simulink model "pll918"  (R2021b)
settings: Solver=VariableStepAuto  StartTime=0.0  StopTime=0.1  RelTol=1e-3
libraries: spsIGBTDiodeLib x6, cstextras x4, spsAlphaBetaZerotodq0Lib x3, slpidlib x3, spsabctoAlphaBetaZeroLib x3, spsThreePhaseSeriesRLCBranchLib x2, spsThreePhaseVIMeasurementLib x2, spsAlphaBetaZerotoabcLib x1, spsGroundLib x1, spsSawtoothGeneratorLib x1, spsDCVoltageSourceLib x1, spsSeriesRLCBranchLib x1
settings Model: Creator=Admin  LastModifiedBy=Admin

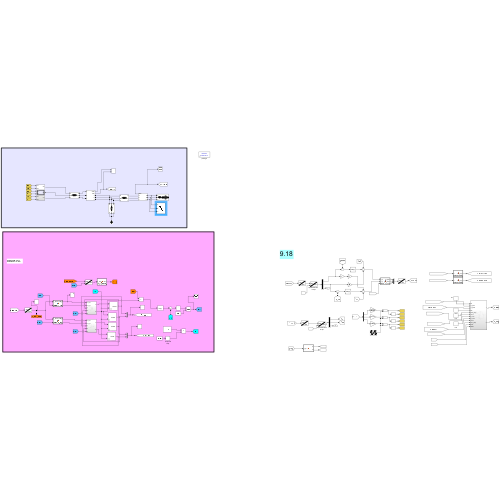
[thumbnail: Simulink's stored preview of the top-level diagram]
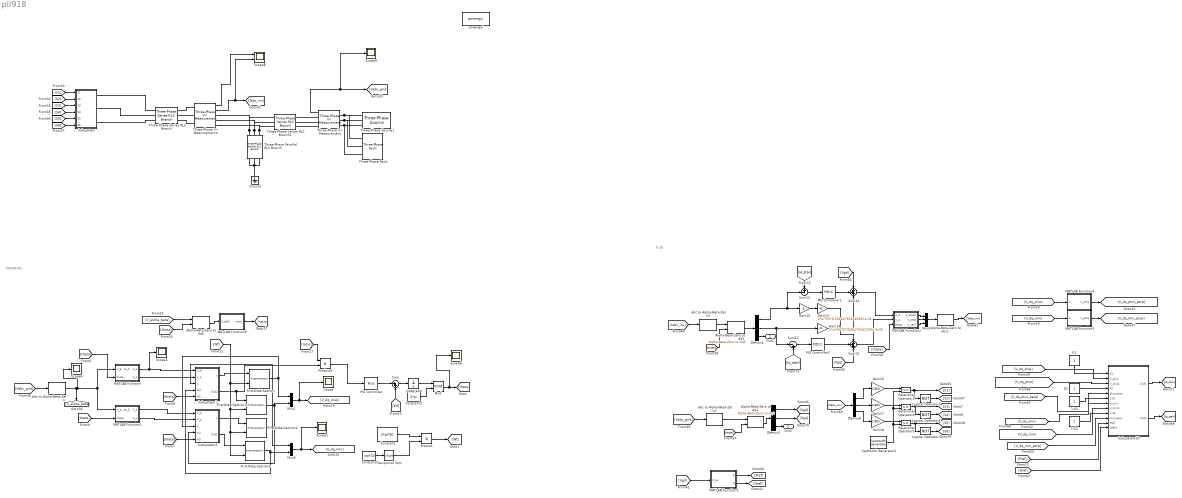
== system pll918 ==
  note: DDSRF-PLL
  note: 9.18
  1-K1 : Constant
  1-K2 : Constant
  Alpha-Beta-Zero to abc1 : spsAlphaBetaZerotoabcLib/Alpha-Beta-Zero to abc
      settings: SourceProductBaseCode=PS
  Alpha-Beta-Zero to dq0 : spsAlphaBetaZerotodq0Lib/Alpha-Beta-Zero to dq0  Alignment=90 degrees behind phase A axis
      settings: SourceProductBaseCode=PS
  Alpha-Beta-Zero to dq1 : spsAlphaBetaZerotodq0Lib/Alpha-Beta-Zero to dq0  Alignment=90 degrees behind phase A axis
      settings: SourceProductBaseCode=PS
  Alpha-Beta-Zero to dq2 : spsAlphaBetaZerotodq0Lib/Alpha-Beta-Zero to dq0  Alignment=90 degrees behind phase A axis
      settings: SourceProductBaseCode=PS
  Constant : Constant  Value=2*pi*50
  Constant1 : Constant  Value=sqrt(2)
  Constant2 : Constant  Value=2*pi
  Demux3 : Demux  Outputs=3
  Demux4 : Demux  Outputs=3
  Demux6 : Demux  Outputs=3
  FirstOrderSection{,1..3} (4 alike) : cstextras/FirstOrderSection  VariantControl=(default)
      settings: SourceProductBaseCode=CT
  Gain13 : Gain  Gain=2*pi*50*6.254627916220947e-05
  Gain14 : Gain  Gain=2*pi*50*6.254627916220947e-05
  Gain15 : Gain  Gain=-1
  Gain16 : Gain  Gain=2/800
  Gain17 : Gain  Gain=2/800
  Gain18 : Gain  Gain=2/800
  Ground : spsGroundLib/Ground  LConnTagsString=a
  Integrator : Integrator
  "K1 " : Constant
  K2 : Constant
  Logical Operator3 : Logic  Operator=NOT  AllPortsSameDT=off  OutDataTypeStr=boolean
  Logical Operator4 : Logic  Operator=NOT  AllPortsSameDT=off  OutDataTypeStr=boolean
  Logical Operator5 : Logic  Operator=NOT  AllPortsSameDT=off  OutDataTypeStr=boolean
  MATLAB Function : MATLAB Function  TreatAsAtomicUnit=on
  MATLAB Function1 : MATLAB Function  TreatAsAtomicUnit=on
  MATLAB Function2 : MATLAB Function  TreatAsAtomicUnit=on
  MATLAB Function3 : MATLAB Function  TreatAsAtomicUnit=on
  MATLAB Function4 : MATLAB Function  TreatAsAtomicUnit=on
  MATLAB Function5 : MATLAB Function  TreatAsAtomicUnit=on
  MATLAB Function8 : MATLAB Function  TreatAsAtomicUnit=on
  Mod : Math  Operator=mod  SaturateOnIntegerOverflow=on
  Mux1 : Mux  Inputs=2
  Mux3 : Mux  Inputs=3
  Mux6 : Mux  Inputs=2
  PID Controller : slpidlib/PID Controller  Controller=PI  Form=Parallel  TimeDomain=Continuous-time  UseExternalTs=off  SampleTime=-1  IntegratorMethod=Forward Euler  FilterMethod=Forward Euler  ControllerParametersSource=internal  P=222.1  I=9e-3  D=0  UseFilter=on  N=100  TunerSelectOption=Transfer Function Based (PID Tuner App)  InitialConditionSource=internal  InitialConditionForIntegrator=0  InitialConditionForFilter=0  DifferentiatorICPrevScaledInput=0  ExternalReset=none  TrackingMode=off  Kt=1  LimitOutput=off  SatLimitsSource=internal  UpperSaturationLimit=inf  LowerSaturationLimit=-inf  LinearizeAsGain=on  AntiWindupMode=none  Kb=1  POutMin=[]  POutMax=[]  IOutMin=[]  IOutMax=[]  DOutMin=[]  DOutMax=[]  NOutMin=[]  NOutMax=[]  SumOutMin=[]  SumOutMax=[]  SaturationOutMin=[]  SaturationOutMax=[]  PParamMin=[]  PParamMax=[]  IParamMin=[]  IParamMax=[]  DParamMin=[]  DParamMax=[]  NParamMin=[]  NParamMax=[]  KbParamMin=[]  KbParamMax=[]  KtParamMin=[]  KtParamMax=[]  KbOutMin=[]  KbOutMax=[]  KtOutMin=[]  KtOutMax=[]  IntegratorOutMin=[]  IntegratorOutMax=[]  FilterOutMin=[]  FilterOutMax=[]  SumI1OutMin=[]  SumI1OutMax=[]  SumI2OutMin=[]  SumI2OutMax=[]  SumI3OutMin=[]  SumI3OutMax=[]  SumI4OutMin=[]  SumI4OutMax=[]  SumDOutMin=[]  SumDOutMax=[]  DifferentiatorOutMin=[]  DifferentiatorOutMax=[]  FilterDiffOutCoefMin=[]  FilterDiffOutCoefMax=[]  ReciprocalOutMin=[]  ReciprocalOutMax=[]  SumDenOutMin=[]  SumDenOutMax=[]  SumNumOutMin=[]  SumNumOutMax=[]  DivideOutMin=[]  DivideOutMax=[]  UdiffTsProdOutMin=[]  UdiffTsProdOutMax=[]  NTsProdOutMin=[]  NTsProdOutMax=[]  UintegralTsProdOutMin=[]  UintegralTsProdOutMax=[]  UngainTsProdOutMin=[]  UngainTsProdOutMax=[]  FilterDenConstantOutDataTypeStr=Inherit: Inherit via back propagation  FilterDenConstantOutMin=[]  FilterDenConstantOutMax=[]  PCopyOutDataTypeStr=Inherit: Inherit via back propagation  PCopyOutMin=[]  PCopyOutMax=[]  NCopyOutDataTypeStr=Inherit: Inherit via back propagation  NCopyOutMin=[]  NCopyOutMax=[]  IntegratorContinuousStateAttributes=''  IntegratorStateMustResolveToSignalObject=off  IntegratorRTWStateStorageClass=Auto  FilterContinuousStateAttributes=''  FilterStateMustResolveToSignalObject=off  FilterRTWStateStorageClass=Auto  ParallelPVariant=InternalParameters  IdealPVariant=Disabled  IVariant=InternalParameters  DVariant=Disabled  IntegratorVariant=Continuous  SatVariant=Disabled  AWVariant=Passthrough  PCopyVariant=Disabled  TRVariant=Disabled  FdbkBlocksVariant=Forward  IdealPFdbkVariant=Disabled  SatFdbkVariant=Disabled  DerivativeFilterVariant=Disabled  NVariant=Disabled  NCopyVariant=Disabled_SignalSpec  FilterICVariant=Disabled  IntegratorICVariant=InternalICs  ExternalResetVariant=Disabled  TRSumVariant=Passthrough  SumFdbkVariant=Disabled  SumVariant=Sum_PI  TsampFilterVariant=InternalTs  TsampNgainVariant=Passthrough  TsampIntegralVariant=Passthrough  ExternalSaturationOutDataTypeStr=Inherit: Same as second input
  PID Controller1 : slpidlib/PID Controller  Controller=PID  Form=Parallel  TimeDomain=Discrete-time  UseExternalTs=off  SampleTime=-1  IntegratorMethod=Forward Euler  FilterMethod=Forward Euler  ControllerParametersSource=internal  P=5  I=1  D=0  UseFilter=on  N=100  TunerSelectOption=Transfer Function Based (PID Tuner App)  InitialConditionSource=internal  InitialConditionForIntegrator=0  InitialConditionForFilter=0  DifferentiatorICPrevScaledInput=0  ExternalReset=none  TrackingMode=off  Kt=1  LimitOutput=off  SatLimitsSource=internal  UpperSaturationLimit=inf  LowerSaturationLimit=-inf  LinearizeAsGain=on  AntiWindupMode=none  Kb=1  POutMin=[]  POutMax=[]  IOutMin=[]  IOutMax=[]  DOutMin=[]  DOutMax=[]  NOutMin=[]  NOutMax=[]  SumOutMin=[]  SumOutMax=[]  SaturationOutMin=[]  SaturationOutMax=[]  PParamMin=[]  PParamMax=[]  IParamMin=[]  IParamMax=[]  DParamMin=[]  DParamMax=[]  NParamMin=[]  NParamMax=[]  KbParamMin=[]  KbParamMax=[]  KtParamMin=[]  KtParamMax=[]  KbOutMin=[]  KbOutMax=[]  KtOutMin=[]  KtOutMax=[]  IntegratorOutMin=[]  IntegratorOutMax=[]  FilterOutMin=[]  FilterOutMax=[]  SumI1OutMin=[]  SumI1OutMax=[]  SumI2OutMin=[]  SumI2OutMax=[]  SumI3OutMin=[]  SumI3OutMax=[]  SumI4OutMin=[]  SumI4OutMax=[]  SumDOutMin=[]  SumDOutMax=[]  DifferentiatorOutMin=[]  DifferentiatorOutMax=[]  FilterDiffOutCoefMin=[]  FilterDiffOutCoefMax=[]  ReciprocalOutMin=[]  ReciprocalOutMax=[]  SumDenOutMin=[]  SumDenOutMax=[]  SumNumOutMin=[]  SumNumOutMax=[]  DivideOutMin=[]  DivideOutMax=[]  UdiffTsProdOutMin=[]  UdiffTsProdOutMax=[]  NTsProdOutMin=[]  NTsProdOutMax=[]  UintegralTsProdOutMin=[]  UintegralTsProdOutMax=[]  UngainTsProdOutMin=[]  UngainTsProdOutMax=[]  FilterDenConstantOutDataTypeStr=Inherit: Inherit via back propagation  FilterDenConstantOutMin=[]  FilterDenConstantOutMax=[]  PCopyOutDataTypeStr=Inherit: Inherit via back propagation  PCopyOutMin=[]  PCopyOutMax=[]  NCopyOutDataTypeStr=Inherit: Inherit via back propagation  NCopyOutMin=[]  NCopyOutMax=[]  IntegratorContinuousStateAttributes=''  IntegratorStateMustResolveToSignalObject=off  IntegratorRTWStateStorageClass=Auto  FilterContinuousStateAttributes=''  FilterStateMustResolveToSignalObject=off  FilterRTWStateStorageClass=Auto  ParallelPVariant=InternalParameters  IdealPVariant=Disabled  IVariant=InternalParameters  DVariant=InternalParameters  IntegratorVariant=Discrete  SatVariant=Disabled  AWVariant=Passthrough  PCopyVariant=Disabled  TRVariant=Disabled  FdbkBlocksVariant=Forward  IdealPFdbkVariant=Disabled  SatFdbkVariant=Disabled  DerivativeFilterVariant=ForwardEulerFilter  NVariant=InternalParameters  NCopyVariant=Disabled  FilterICVariant=InternalICsFilter  IntegratorICVariant=InternalICs  ExternalResetVariant=Disabled  TRSumVariant=Passthrough  SumFdbkVariant=Disabled  SumVariant=Sum_PID  TsampFilterVariant=InternalTs  TsampNgainVariant=Passthrough  TsampIntegralVariant=Passthrough  ExternalSaturationOutDataTypeStr=Inherit: Same as second input
  PID Controller2 : slpidlib/PID Controller  Controller=PID  Form=Parallel  TimeDomain=Discrete-time  UseExternalTs=off  SampleTime=-1  IntegratorMethod=Forward Euler  FilterMethod=Forward Euler  ControllerParametersSource=internal  P=5  I=1  D=0  UseFilter=on  N=100  TunerSelectOption=Transfer Function Based (PID Tuner App)  InitialConditionSource=internal  InitialConditionForIntegrator=0  InitialConditionForFilter=0  DifferentiatorICPrevScaledInput=0  ExternalReset=none  TrackingMode=off  Kt=1  LimitOutput=off  SatLimitsSource=internal  UpperSaturationLimit=inf  LowerSaturationLimit=-inf  LinearizeAsGain=on  AntiWindupMode=none  Kb=1  POutMin=[]  POutMax=[]  IOutMin=[]  IOutMax=[]  DOutMin=[]  DOutMax=[]  NOutMin=[]  NOutMax=[]  SumOutMin=[]  SumOutMax=[]  SaturationOutMin=[]  SaturationOutMax=[]  PParamMin=[]  PParamMax=[]  IParamMin=[]  IParamMax=[]  DParamMin=[]  DParamMax=[]  NParamMin=[]  NParamMax=[]  KbParamMin=[]  KbParamMax=[]  KtParamMin=[]  KtParamMax=[]  KbOutMin=[]  KbOutMax=[]  KtOutMin=[]  KtOutMax=[]  IntegratorOutMin=[]  IntegratorOutMax=[]  FilterOutMin=[]  FilterOutMax=[]  SumI1OutMin=[]  SumI1OutMax=[]  SumI2OutMin=[]  SumI2OutMax=[]  SumI3OutMin=[]  SumI3OutMax=[]  SumI4OutMin=[]  SumI4OutMax=[]  SumDOutMin=[]  SumDOutMax=[]  DifferentiatorOutMin=[]  DifferentiatorOutMax=[]  FilterDiffOutCoefMin=[]  FilterDiffOutCoefMax=[]  ReciprocalOutMin=[]  ReciprocalOutMax=[]  SumDenOutMin=[]  SumDenOutMax=[]  SumNumOutMin=[]  SumNumOutMax=[]  DivideOutMin=[]  DivideOutMax=[]  UdiffTsProdOutMin=[]  UdiffTsProdOutMax=[]  NTsProdOutMin=[]  NTsProdOutMax=[]  UintegralTsProdOutMin=[]  UintegralTsProdOutMax=[]  UngainTsProdOutMin=[]  UngainTsProdOutMax=[]  FilterDenConstantOutDataTypeStr=Inherit: Inherit via back propagation  FilterDenConstantOutMin=[]  FilterDenConstantOutMax=[]  PCopyOutDataTypeStr=Inherit: Inherit via back propagation  PCopyOutMin=[]  PCopyOutMax=[]  NCopyOutDataTypeStr=Inherit: Inherit via back propagation  NCopyOutMin=[]  NCopyOutMax=[]  IntegratorContinuousStateAttributes=''  IntegratorStateMustResolveToSignalObject=off  IntegratorRTWStateStorageClass=Auto  FilterContinuousStateAttributes=''  FilterStateMustResolveToSignalObject=off  FilterRTWStateStorageClass=Auto  ParallelPVariant=InternalParameters  IdealPVariant=Disabled  IVariant=InternalParameters  DVariant=InternalParameters  IntegratorVariant=Discrete  SatVariant=Disabled  AWVariant=Passthrough  PCopyVariant=Disabled  TRVariant=Disabled  FdbkBlocksVariant=Forward  IdealPFdbkVariant=Disabled  SatFdbkVariant=Disabled  DerivativeFilterVariant=ForwardEulerFilter  NVariant=InternalParameters  NCopyVariant=Disabled  FilterICVariant=InternalICsFilter  IntegratorICVariant=InternalICs  ExternalResetVariant=Disabled  TRSumVariant=Passthrough  SumFdbkVariant=Disabled  SumVariant=Sum_PID  TsampFilterVariant=InternalTs  TsampNgainVariant=Passthrough  TsampIntegralVariant=Passthrough  ExternalSaturationOutDataTypeStr=Inherit: Same as second input
  Product : Product
  Product9 : Product
  Reciprocal Sqrt : Sqrt  Operator=rSqrt  IntermediateResultsDataTypeStr=double  SaturateOnIntegerOverflow=on
  Relational Operator3 : RelationalOperator  OutDataTypeStr=boolean  RndMeth=Simplest
  Relational Operator4 : RelationalOperator  OutDataTypeStr=boolean  RndMeth=Simplest
  Relational Operator5 : RelationalOperator  OutDataTypeStr=boolean  RndMeth=Simplest
  Sawtooth Generator2 : spsSawtoothGeneratorLib/Sawtooth Generator  Freq=120e3  Phase=180  Ts=0
  Scope{,1,4..6,9} (6 alike) : Scope
  Scope8 : Scope  NumInputPorts=2
  Subsystem : Subsystem
  Subsystem1 : Subsystem
  Subsystem10 : Subsystem
  Subsystem3 : Subsystem
  Sum : Sum  Inputs=|++
  Sum12 : Sum  Inputs=+-|
  Sum13 : Sum  Inputs=|-+
  Sum14 : Sum  Inputs=+++
  Sum15 : Sum  Inputs=+++
  Three-Phase Parallel RLC Branch : spsThreePhaseParallelRLCBranchLib/Three-Phase Parallel RLC Branch  LConnTagsString=A|B|C  RConnTagsString=A|B|C  BranchType=C  Resistance=1  Inductance=1e-3  Capacitance=4.22171e-05  Measurements=None
      settings: SourceProductBaseCode=PS
  Three-Phase Series RLC Branch : spsThreePhaseSeriesRLCBranchLib/Three-Phase Series RLC Branch  LConnTagsString=A|B|C  RConnTagsString=A|B|C  BranchType=L  Resistance=1  Inductance=25.6e-06  Capacitance=1e-6  Measurements=None
  Three-Phase Series RLC Branch1 : spsThreePhaseSeriesRLCBranchLib/Three-Phase Series RLC Branch  LConnTagsString=A|B|C  RConnTagsString=A|B|C  BranchType=L  Resistance=1  Inductance=5e-06  Capacitance=1e-6  Measurements=None
  Three-Phase V-I Measurement : spsThreePhaseVIMeasurementLib/Three-Phase V-I Measurement  VoltageMeasurement=phase-to-ground  SetLabelV=off  LabelV=Vabc  Vpu=off  VpuLL=off  CurrentMeasurement=no  SetLabelI=off  LabelI=Iabc  Ipu=off  Pbase=100e6  Vbase=400  OutputType=Complex  PhasorSimulation=off  PSBequivalent=0
  Three-Phase V-I Measurement4 : spsThreePhaseVIMeasurementLib/Three-Phase V-I Measurement  VoltageMeasurement=phase-to-ground  SetLabelV=off  LabelV=Vabc  Vpu=on  VpuLL=off  CurrentMeasurement=yes  SetLabelI=off  LabelI=Iabc  Ipu=off  Pbase=100e6  Vbase=400  OutputType=Complex  PhasorSimulation=off  PSBequivalent=0
  Three-Phase Fault : spsThreePhaseFaultLib/Three-Phase Fault  InitialStates=0  FaultA=on  FaultB=on  FaultC=off  GroundFault=off  SwitchTimes="[0.03  0.04]"  External=off  SwitchStatus=NaN  FaultResistance=0.001  GroundResistance=0.01  SnubberResistance=1e6  SnubberCapacitance=inf  Measurements=Fault voltages
  Three-Phase Source1 : spsThreePhaseSourceLib/Three-Phase Source  InternalConnection=Yg  VoltagePhases=off  Voltage=400  PhaseAngle=0  Voltage_phases=[25e3 25e3 25e3]/sqrt(3)  PhaseAngles_phases=[0 -120 +120]  Frequency=50  NonIdealSource=on  SpecifyImpedance=off  Resistance=(50e-6*2*pi*50)/2  Inductance=50e-6  ShortCircuitLevel=160e3  BaseVoltage=400/sqrt(3)  XRratio=10  BusType=PQ  Pref=160e3  Qref=50000  Prefabc=[10e3, 10e3, 10e3]  Qrefabc=[0, 0, 0]  Qmin=-inf  Qmax=inf
  abc to Alpha-Beta-Zero : spsabctoAlphaBetaZeroLib/abc to Alpha-Beta-Zero
      settings: SourceProductBaseCode=PS
  abc to Alpha-Beta-Zero2 : spsabctoAlphaBetaZeroLib/abc to Alpha-Beta-Zero
      settings: SourceProductBaseCode=PS
  abc to Alpha-Beta-Zero3 : spsabctoAlphaBetaZeroLib/abc to Alpha-Beta-Zero
      settings: SourceProductBaseCode=PS
  powergui : spspowerguiLib/powergui  Priority=1  SimulationMode=Discrete  SampleTime=6.024e-05  frequency=60  Iterations=50  frequencyindice=50  Pbase=100e6  ErrMax=1e-4  UnitsV=kV  UnitsW=MW  buscounter=0  FunctionMessages=off  echomessages=off  EnableUseOfTLC=off  CurrentSourceSwitches=off  DisableSnubberDevices=off  DisableRonSwitches=off  DisableVfSwitches=off  DisplayEquations=off  AutomaticDiscreteSolvers=off  SolverType=Tustin/Backward Euler (TBE)  Interpol=off  ExternalGateDelay=off  methode=off  Ts=100  x0status=blocks  SPID=on  SwTol=0  HookPort=off  NonlinearTolerance=1e-4  nMaxIteration=100  ContinueOnMaxIteration=off  RestoreLinks=warning  ResistiveCurrentMeasurement=off  Frange=[0:2:500]  Ylog=off  Xlog=on  ShowGrid=off  save=off  variable=ZData  structure=0  ZoomFFT=off  StartTime=0.0  cycles=1  DisplayStyle=1  fundamental=60  FreqAxis=off  MaxFrequency=1000  frequencyindicesteady=1  RmsSteady=1  display=off
  Out1 : Outport
  Out2 : Outport  Port=2
  wires:
  [S6] -> Subsystem/6(S6)
  Three-Phase V-I Measurement/1 -> Scope9/1, [Vabc_grid]
  [S1] -> Subsystem/1(S1)
  Three-Phase V-I Measurement4/1 -> Scope8/1
  [S2] -> Subsystem/2(S2)
  [S4] -> Subsystem/4(S4)
  [S5] -> Subsystem/5(S5)
  [S3] -> Subsystem/3(S3)
  Three-Phase V-I Measurement4/2 -> Scope8/2, [Iabc_inv]
  Integrator/1 -> Mod/1
  Constant1/1 -> Reciprocal Sqrt/1
  MATLAB Function1/1(V_d) -> Subsystem3/1(V_d)
  MATLAB Function8/1(ratio) -> [ratio]
  MATLAB Function1/2(V_q) -> Subsystem3/2(V_q)
  [theta] -> Alpha-Beta-Zero to dq0/2
  Product9/1 -> PID Controller/1
  MATLAB Function/2(V_q) -> Subsystem1/2(V_q)
  Product/1 -> [Wf]
  Mod/1 -> Scope6/1, [theta]
  [V_alpha_beta] -> Alpha-Beta-Zero to dq0/1
  FirstOrderSection/1 -> Mux1/1, Subsystem3/3(y)
  Alpha-Beta-Zero to dq0/1 -> MATLAB Function8/1(V_dq0)
  Constant/1 -> Product/1
  [Wf] -> Sum/2
  PID Controller/1 -> Sum/1
  Reciprocal Sqrt/1 -> Product/2
  [theta] -> Subsystem1/5(In5)
  [Vabc_grid] -> abc to Alpha-Beta-Zero/1
  Subsystem3/2(Out2) -> FirstOrderSection3/1
  FirstOrderSection1/1 -> Mux1/2, Subsystem3/4(In4)
  FirstOrderSection2/1 -> Mux6/1, Subsystem1/3(y)
  abc to Alpha-Beta-Zero/1 -> MATLAB Function1/1(V_alpha_beta_0), MATLAB Function/1(V_alpha_beta_0), Scope4/1, [V_alpha_beta]
  Constant2/1 -> Mod/2
  [ratio] -> Product9/1
  Sum/1 -> Integrator/1
  Mux6/1 -> Scope1/1, [V_dq_min]
  Subsystem3/1(u) -> FirstOrderSection2/1
  Subsystem1/2(Out2) -> FirstOrderSection1/1, Product9/2
  [Wf] -> FirstOrderSection/2, FirstOrderSection3/2, FirstOrderSection2/2, FirstOrderSection1/2
  [theta] -> MATLAB Function1/2(theta)
  Subsystem1/1(u) -> FirstOrderSection/1
  [theta] -> Subsystem3/5(In5)
  [theta] -> MATLAB Function/2(theta)
  FirstOrderSection3/1 -> Subsystem1/4(In4), Mux6/2
  MATLAB Function/1(V_d) -> Scope5/1, Subsystem1/1(V_d)
  MATLAB Function2/3(V_zero) -> Mux3/3
  Relational Operator4/1 -> Logical Operator4/1, [S3]
  Sum14/1 -> MATLAB Function2/1(V_d)
  Sum15/1 -> MATLAB Function2/2(V_q)
  Sawtooth Generator2/1 -> Relational Operator3/2, Relational Operator4/2, Relational Operator5/2
  Demux4/1 -> Gain15/1, Sum12/2
  Demux6/3 -> Gain18/1
  [V_dq_plus_perp] -> Subsystem10/5(plus_perp)
  Gain16/1 -> Relational Operator3/1
  [Vgq] -> Sum15/3
  PID Controller2/1 -> Sum15/2
  [Id_star] -> Sum12/1
  Demux4/3 -> Out1/1
  Sum12/1 -> PID Controller1/1
  Demux4/2 -> Sum13/1, Gain14/1
  PID Controller1/1 -> Sum14/2
  MATLAB Function3/1(P) -> [Pref]
  Gain17/1 -> Relational Operator4/1
  abc to Alpha-Beta-Zero3/1 -> Alpha-Beta-Zero to dq2/1
  Demux3/2 -> [Vgq]
  Gain15/1 -> Gain13/1
  [Vabc_inv] -> Demux6/1
  MATLAB Function4/1(V_perp) -> [V_dq_plus_perp]
  1-K1/1 -> Subsystem10/6(1-K1)
  1-K2/1 -> Subsystem10/9(1-K2)
  Demux3/1 -> [Vgd]
  "K1 "/1 -> Subsystem10/1(K1)
  Logical Operator4/1 -> [S4]
  MATLAB Function3/2(Q) -> [Qref]
  [V_dq_min] -> Subsystem10/7(V_min)
  [Vabc_grid] -> abc to Alpha-Beta-Zero2/1
  Sum13/1 -> PID Controller2/1
  Relational Operator3/1 -> [S1], Logical Operator3/1
  MATLAB Function2/2(V_beta) -> Mux3/2
  K2/1 -> Subsystem10/4(K2)
  [V_dq_plus] -> MATLAB Function4/1(V)
  [V_dq_min_perp] -> Subsystem10/10(min_perp)
  Gain14/1 -> Sum14/3
  [Qref] -> Subsystem10/12(Qref1)
  Alpha-Beta-Zero to dq2/1 -> Demux4/1
  Gain13/1 -> Sum15/1
  Demux3/3 -> Out2/1
  [Pref] -> Subsystem10/11(Pref)
  [theta] -> Alpha-Beta-Zero to dq2/2
  MATLAB Function5/1(V_perp) -> [V_dq_min_perp]
  Demux6/2 -> Gain17/1
  Logical Operator3/1 -> [S2]
  [Iq_star] -> Sum13/2
  abc to Alpha-Beta-Zero2/1 -> Alpha-Beta-Zero to dq1/1
  [theta] -> Alpha-Beta-Zero to dq1/2
  Alpha-Beta-Zero to dq1/1 -> Demux3/1
  [V_dq_min] -> Subsystem10/8(V_min1)
  Demux6/1 -> Gain16/1
  [Vgd] -> Sum14/1
  Logical Operator5/1 -> [S6]
  Gain18/1 -> Relational Operator5/1
  [theta] -> MATLAB Function2/3(theta)
  Relational Operator5/1 -> [S5], Logical Operator5/1
  [Iabc_inv] -> abc to Alpha-Beta-Zero3/1
  Subsystem10/1(Out1) -> [Id_star]
  Subsystem10/2(Out2) -> [Iq_star]
  MATLAB Function2/1(V_alpha) -> Mux3/1
  [V_dq_plus] -> Subsystem10/2(V_plus)
  Mux3/1 -> Alpha-Beta-Zero to abc1/1
  [V_dq_plus] -> Subsystem10/3(V_plus1)
  Alpha-Beta-Zero to abc1/1 -> [Vabc_inv]
  [Vgd] -> MATLAB Function3/1(V_pu)
  [V_dq_min] -> MATLAB Function5/1(V)
  Mux1/1 -> Scope/1, [V_dq_plus]
  connections:
  Three-Phase V-I Measurement/LConn2 -- Three-Phase Source1/RConn2 -- Three-Phase Fault/LConn2
  Three-Phase V-I Measurement/LConn3 -- Three-Phase Source1/RConn3 -- Three-Phase Fault/LConn3
  Three-Phase Parallel RLC Branch/LConn3 -- Three-Phase V-I Measurement4/RConn3 -- Three-Phase Series RLC Branch1/LConn3
  Three-Phase Parallel RLC Branch/LConn1 -- Three-Phase V-I Measurement4/RConn1 -- Three-Phase Series RLC Branch1/LConn1
  Three-Phase V-I Measurement/LConn1 -- Three-Phase Source1/RConn1 -- Three-Phase Fault/LConn1
  Three-Phase Parallel RLC Branch/RConn1 -- Three-Phase Parallel RLC Branch/RConn2 -- Ground/LConn1 -- Three-Phase Parallel RLC Branch/RConn3
  Three-Phase Parallel RLC Branch/LConn2 -- Three-Phase V-I Measurement4/RConn2 -- Three-Phase Series RLC Branch1/LConn2
  Three-Phase V-I Measurement/RConn3 -- Three-Phase Series RLC Branch1/RConn3
  Subsystem/RConn3 -- Three-Phase Series RLC Branch/LConn3
  Subsystem/RConn1 -- Three-Phase Series RLC Branch/LConn1
  Three-Phase V-I Measurement/RConn1 -- Three-Phase Series RLC Branch1/RConn1
  Three-Phase V-I Measurement4/LConn2 -- Three-Phase Series RLC Branch/RConn2
  Subsystem/RConn2 -- Three-Phase Series RLC Branch/LConn2
  Three-Phase V-I Measurement4/LConn1 -- Three-Phase Series RLC Branch/RConn1
  Three-Phase V-I Measurement/RConn2 -- Three-Phase Series RLC Branch1/RConn2
  Three-Phase V-I Measurement4/LConn3 -- Three-Phase Series RLC Branch/RConn3

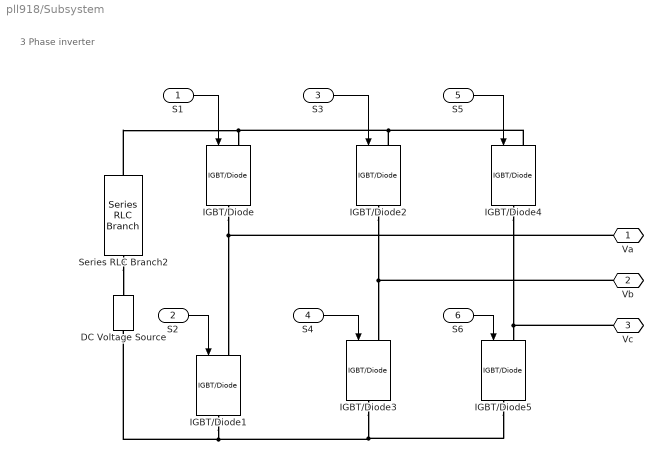
== system pll918/Subsystem ==
  note: 3 Phase inverter
  S1 : Inport
  S2 : Inport  Port=2
  S3 : Inport  Port=3
  S4 : Inport  Port=4
  S5 : Inport  Port=5
  S6 : Inport  Port=6
  DC Voltage Source : spsDCVoltageSourceLib/DC Voltage Source  Amplitude=800  Measurements=None
  IGBT/Diode{,1..5} (6 alike) : spsIGBTDiodeLib/IGBT//Diode  Ron=0.01  Rs=10  Cs=0.1e-6  Measurements=off
  Series RLC Branch2 : spsSeriesRLCBranchLib/Series RLC Branch  LConnTagsString=__new0  RConnTagsString=__new0  BranchType=R  Resistance=0.01  Inductance=1e-3  SetiL0=off  InitialCurrent=0  Capacitance=1e-6  Setx0=off  InitialVoltage=0  Measurements=None
  Va : PMIOPort  Side=Right
  Vb : PMIOPort  Port=2  Side=Right
  Vc : PMIOPort  Port=3  Side=Right
  wires:
  S1/1 -> IGBT/Diode/1
  S2/1 -> IGBT/Diode1/1
  S4/1 -> IGBT/Diode3/1
  S5/1 -> IGBT/Diode4/1
  S3/1 -> IGBT/Diode2/1
  S6/1 -> IGBT/Diode5/1
  connections:
  IGBT/Diode2/RConn1 -- Vb/RConn1 -- IGBT/Diode3/LConn1
  IGBT/Diode/RConn1 -- Va/RConn1 -- IGBT/Diode1/LConn1
  IGBT/Diode2/LConn1 -- Series RLC Branch2/RConn1 -- IGBT/Diode/LConn1 -- IGBT/Diode4/LConn1
  IGBT/Diode3/RConn1 -- IGBT/Diode1/RConn1 -- DC Voltage Source/LConn1 -- IGBT/Diode5/RConn1
  IGBT/Diode4/RConn1 -- Vc/RConn1 -- IGBT/Diode5/LConn1
  Series RLC Branch2/LConn1 -- DC Voltage Source/RConn1

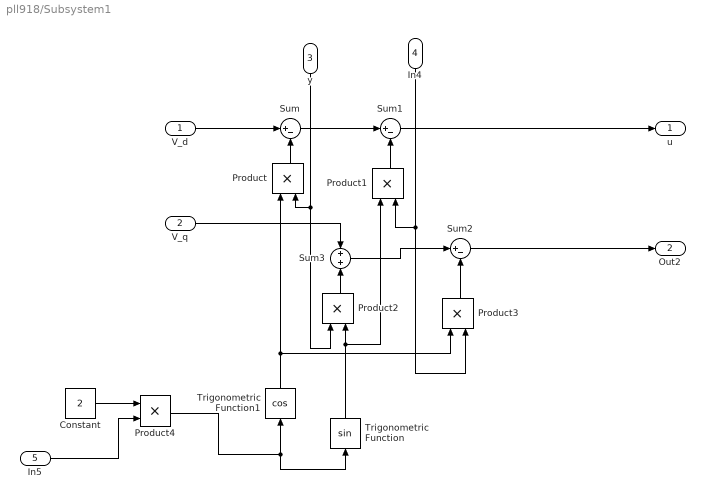
== system pll918/Subsystem1 ==
  V_d : Inport
  V_q : Inport  Port=2
  y : Inport  Port=3
  In4 : Inport  Port=4
  In5 : Inport  Port=5
  Constant : Constant  Value=2
  Product{,1..4} (5 alike) : Product
  Sum : Sum  Inputs=|+-
  Sum1 : Sum  Inputs=|+-
  Sum2 : Sum  Inputs=|+-
  Sum3 : Sum
  Trigonometric Function : Trigonometry
  Trigonometric Function1 : Trigonometry  Operator=cos
  u : Outport
  Out2 : Outport  Port=2
  wires:
  Product2/1 -> Sum3/2
  Trigonometric Function1/1 -> Product/1, Product3/1
  In4/1 -> Product1/2, Product3/2
  Sum1/1 -> u/1
  Product/1 -> Sum/2
  V_d/1 -> Sum/1
  Product1/1 -> Sum1/2
  V_q/1 -> Sum3/1
  Sum3/1 -> Sum2/1
  Sum/1 -> Sum1/1
  Trigonometric Function/1 -> Product1/1, Product2/2
  Product3/1 -> Sum2/2
  Product4/1 -> Trigonometric Function/1, Trigonometric Function1/1
  y/1 -> Product2/1, Product/2
  Sum2/1 -> Out2/1
  Constant/1 -> Product4/1
  In5/1 -> Product4/2

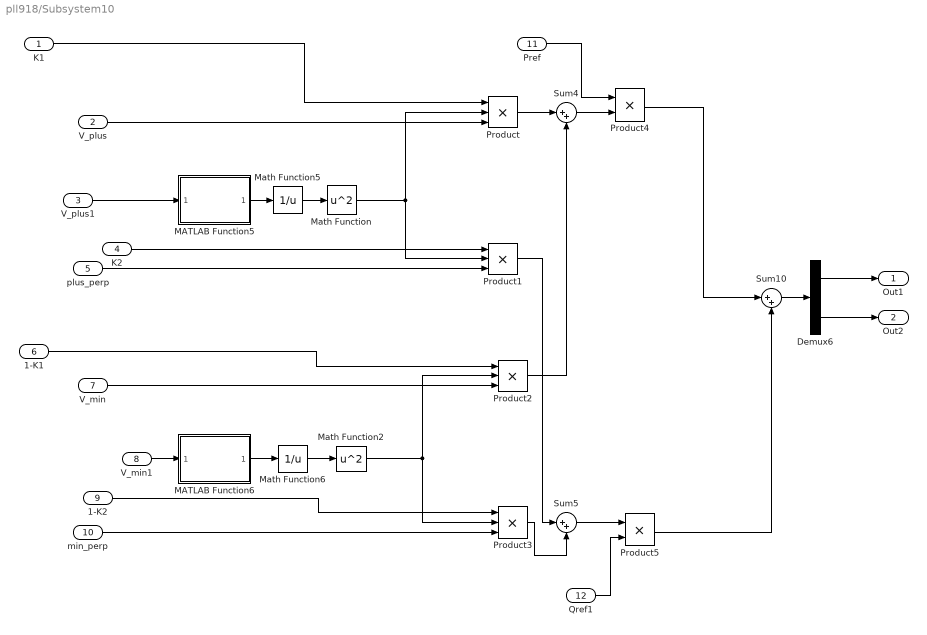
== system pll918/Subsystem10 ==
  K1 : Inport
  V_plus : Inport  Port=2
  V_plus1 : Inport  Port=3
  K2 : Inport  Port=4
  plus_perp : Inport  Port=5
  1-K1 : Inport  Port=6
  V_min : Inport  Port=7
  V_min1 : Inport  Port=8
  1-K2 : Inport  Port=9
  min_perp : Inport  Port=10
  Pref : Inport  Port=11
  Qref1 : Inport  Port=12
  Demux6 : Demux  Outputs=2
  MATLAB Function5 : MATLAB Function  TreatAsAtomicUnit=on
  MATLAB Function6 : MATLAB Function  TreatAsAtomicUnit=on
  Math Function : Math  Operator=square  SaturateOnIntegerOverflow=on
  Math Function2 : Math  Operator=square  SaturateOnIntegerOverflow=on
  Math Function5 : Math  Operator=reciprocal  SaturateOnIntegerOverflow=on
  Math Function6 : Math  Operator=reciprocal  SaturateOnIntegerOverflow=on
  Product{,1..3} (4 alike) : Product  Inputs=3
  Product4 : Product
  Product5 : Product
  Sum10 : Sum  Inputs=|++
  Sum4 : Sum  Inputs=|++
  Sum5 : Sum  Inputs=|++
  Out1 : Outport
  Out2 : Outport  Port=2
  wires:
  MATLAB Function5/1(v_norm_squared) -> Math Function5/1
  Product3/1 -> Sum5/2
  Math Function6/1 -> Math Function2/1
  Math Function2/1 -> Product2/2, Product3/2
  min_perp/1 -> Product3/3
  Math Function/1 -> Product1/2, Product/2
  Sum5/1 -> Product5/1
  Sum4/1 -> Product4/2
  Product/1 -> Sum4/1
  Product5/1 -> Sum10/2
  K2/1 -> Product1/1
  Demux6/2 -> Out2/1
  1-K1/1 -> Product2/1
  Product4/1 -> Sum10/1
  MATLAB Function6/1(v_norm_squared) -> Math Function6/1
  V_min/1 -> Product2/3
  Product1/1 -> Sum5/1
  Math Function5/1 -> Math Function/1
  Product2/1 -> Sum4/2
  V_min1/1 -> MATLAB Function6/1(V_alpha_beta)
  V_plus1/1 -> MATLAB Function5/1(V_alpha_beta)
  Sum10/1 -> Demux6/1
  Qref1/1 -> Product5/2
  V_plus/1 -> Product/3
  plus_perp/1 -> Product1/3
  1-K2/1 -> Product3/1
  K1/1 -> Product/1
  Demux6/1 -> Out1/1
  Pref/1 -> Product4/1

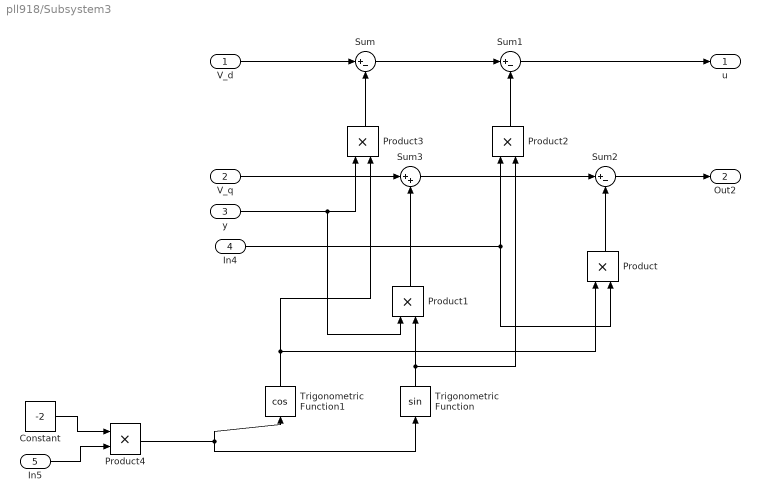
== system pll918/Subsystem3 ==
  V_d : Inport
  V_q : Inport  Port=2
  y : Inport  Port=3
  In4 : Inport  Port=4
  In5 : Inport  Port=5
  Constant : Constant  Value=-2
  Product{,1..4} (5 alike) : Product
  Sum : Sum  Inputs=|+-
  Sum1 : Sum  Inputs=|+-
  Sum2 : Sum  Inputs=|+-
  Sum3 : Sum  Inputs=|++
  Trigonometric Function : Trigonometry
  Trigonometric Function1 : Trigonometry  Operator=cos
  u : Outport
  Out2 : Outport  Port=2
  wires:
  In5/1 -> Product4/2
  Trigonometric Function/1 -> Product2/2, Product1/2
  y/1 -> Product1/1, Product3/1
  Sum/1 -> Sum1/1
  V_q/1 -> Sum3/1
  In4/1 -> Product2/1, Product/2
  Sum3/1 -> Sum2/1
  Constant/1 -> Product4/1
  V_d/1 -> Sum/1
  Product1/1 -> Sum3/2
  Product4/1 -> Trigonometric Function1/1, Trigonometric Function/1
  Product3/1 -> Sum/2
  Sum2/1 -> Out2/1
  Trigonometric Function1/1 -> Product/1, Product3/2
  Sum1/1 -> u/1
  Product/1 -> Sum2/2
  Product2/1 -> Sum1/2

== matlab function pll918/MATLAB Function1 ==
  data: V_alpha_beta_0 input; V_d output; theta input; V_q output
function [V_d, V_q] = calculate_dq(V_alpha_beta_0, theta)
    % Inputs:
    % V_alpha_beta_0 - a 3x1 vector [V_alpha; V_beta; V_0]
    % theta - Angle in radians for transformation (theta')

    % Extract V_alpha and V_beta from the input vector
    V_alpha = V_alpha_beta_0(1);
    V_beta = V_alpha_beta_0(2);
    % Ignore V_0 as it does not affect the dq transformation
    % V_0 = V_alpha_beta_0(3); % Not used in the dq transformation

    % Calculate cos and sin of theta
    cos_theta = cos(theta);
    sin_theta = sin(theta);

    % Define the transformation matrix T_dq
    T_dq = [cos_theta, -sin_theta;
            sin_theta, cos_theta];
    
    % Calculate the dq components
    V_dq = T_dq * [V_alpha; V_beta];
    
    % Extract V_d and V_q
    V_d = V_dq(1);
    V_q = V_dq(2);
end

== matlab function pll918/MATLAB Function ==
  data: V_alpha_beta_0 input; V_d output; theta input; V_q output
function [V_d, V_q] = calculate_dq(V_alpha_beta_0, theta)
    % Inputs:
    % V_alpha_beta_0 - a 3x1 vector [V_alpha; V_beta; V_0]
    % theta - Angle in radians for transformation (theta')

    % Extract V_alpha and V_beta from the input vector
    V_alpha = V_alpha_beta_0(1);
    V_beta = V_alpha_beta_0(2);
    % Ignore V_0 as it does not affect the dq transformation
    % V_0 = V_alpha_beta_0(3); % Not used in the dq transformation

    % Calculate cos and sin of theta
    cos_theta = cos(theta);
    sin_theta = sin(theta);

    % Define the transformation matrix T_dq
    T_dq = [cos_theta, sin_theta;
            -sin_theta, cos_theta];
    
    % Calculate the dq components
    V_dq = T_dq * [V_alpha; V_beta];
    
    % Extract V_d and V_q
    V_d = V_dq(1);
    V_q = V_dq(2);
end

== matlab function pll918/MATLAB Function2 ==
  data: V_d input; V_alpha output; V_q input; theta input; V_beta output; V_zero output
function [V_alpha, V_beta, V_zero] = dq_to_alpha_beta_zero(V_d, V_q, theta)
    % dq_to_alpha_beta_zero: Converts V_d, V_q to V_alpha, V_beta, and V_zero
    %
    % Inputs:
    %   V_d    - Direct-axis voltage component
    %   V_q    - Quadrature-axis voltage component
    %   theta  - Angle of the rotating frame (in radians)
    %
    % Outputs:
    %   V_alpha - Alpha-axis (stationary) voltage component
    %   V_beta  - Beta-axis (stationary) voltage component
    %   V_zero  - Zero-sequence voltage component (typically zero for balanced systems)

    % Compute V_alpha and V_beta using the inverse Park transformation
    V_alpha = V_d * cos(theta) - V_q * sin(theta);
    V_beta  = V_d * sin(theta) + V_q * cos(theta);

    % Compute V_zero (zero-sequence component)
    V_zero = 0;  % Set to zero if there's no zero-sequence component in the system
end

== matlab function pll918/MATLAB Function8 ==
  data: V_dq0 input; ratio output
function ratio  = calculate_magnitude_phase(V_dq0)
    % Inputs:
    % V_dq0 - a 3x1 vector [V_d; V_q; V_0]

    % Extract V_d and V_q from the input vector
    V_d = V_dq0(1);
    V_q = V_dq0(2);
    % V_0 = V_dq0(3); % Not used in magnitude and phase calculation

    % Calculate the magnitude (d)
    magnitude = sqrt(V_d^2 + V_q^2);

    % Calculate the phase angle (q) in radians
    %phase = atan2(V_q, V_d); % atan2 is used for correct quadrant detection

    % Calculate q / sqrt(d^2 + q^2)
    if magnitude ~= 0
        ratio = V_q / magnitude;
    else
        ratio = 0; % Handle the case where the magnitude is zero to avoid division by zero
    end
end

== matlab function pll918/MATLAB Function3 ==
  data: V_pu input; P output; Q output
function [P, Q] = PowerControlLogic(V_pu)
       % Constants
       V_high_threshold = 0.85;  % Upper voltage threshold
       V_low_threshold = 0.4;   % Lower voltage threshold
       S_total = 160;            % Total apparent power (kVA)
       
       % Power Injection Logic
       if V_pu >= V_high_threshold
           % Only active power
           P = S_total;
           Q = 0;
       elseif V_pu <= V_low_threshold
           % Only reactive power
           P = 0;
           Q = S_total;
       else
           % Linear interpolation between thresholds
           power_ratio = (V_high_threshold - V_pu) / ...
                         (V_high_threshold - V_low_threshold);
           
           P = S_total * (1 - power_ratio);
           Q = S_total * power_ratio;
       end
   end

== matlab function pll918/MATLAB Function4 ==
  data: V input; V_perp output
function V_perp = calculatePerpendicular(V)
    % V הוא וקטור דו-ממדי עם שני רכיבים, למשל [V_alpha; V_beta] או [V_d; V_q]
    V1 = V(1);  % הרכיב הראשון של הווקטור (למשל V_alpha או V_d)
    V2 = V(2);  % הרכיב השני של הווקטור (למשל V_beta או V_q)
    
    % חישוב הרכיב הניצב
    V_perp = [-V2; V1];
end

== matlab function pll918/MATLAB Function5 ==
  data: V input; V_perp output
function V_perp = calculatePerpendicular(V)
    % V הוא וקטור דו-ממדי עם שני רכיבים, למשל [V_alpha; V_beta] או [V_d; V_q]
    V1 = V(1);  % הרכיב הראשון של הווקטור (למשל V_alpha או V_d)
    V2 = V(2);  % הרכיב השני של הווקטור (למשל V_beta או V_q)
    
    % חישוב הרכיב הניצב
    V_perp = [-V2; V1];
end

== matlab function pll918/Subsystem10/MATLAB Function5 ==
  data: V_alpha_beta input; v_norm_squared output
function v_norm_squared = calculateNormSquared(V_alpha_beta)
    v_norm_squared = V_alpha_beta(1)^2 + V_alpha_beta(2)^2;
    if v_norm_squared == 0
        v_norm_squared = NaN;
    end
end

== matlab function pll918/Subsystem10/MATLAB Function6 ==
  data: V_alpha_beta input; v_norm_squared output
function v_norm_squared = calculateNormSquared(V_alpha_beta)
    v_norm_squared = V_alpha_beta(1)^2 + V_alpha_beta(2)^2;
    if v_norm_squared == 0
        v_norm_squared = NaN;
    end
end
